simulink model "generic_Truck_And_Trailer"  (R2025a)
settings: Solver=VariableStepAuto  StartTime=0.0  StopTime=350  FixedStep=0.01  MaxStep=0.001  RelTol=1e-3  EnableMultiTasking=on
libraries: TruckMaker4SL x250, simulink x1
(part 10 of 11)

== matlab function generic_Truck_And_Trailer/TruckMaker/Subsystem1/ONE_TRACK_MODEL_TRACTOR_UKF/UKF_ONE_TRACK_TRUCK_AND_TRAILER_WORKING_MODEL  ==
  data: z input; u input; xhat output; Q input; R input; Ts input; P output; dxdt output; innovation output; K_out output; S_out output; z_pred_out output; truck_Ff output; truck_Fr output; trailer_v_hitch output; data input; trailer_v_axle output; trailer_F_hitch output; trailer_F_tire output; truck_v_hitch output
function [xhat, P, dxdt, innovation, K_out, S_out, z_pred_out,truck_Ff,truck_Fr, trailer_v_hitch,trailer_v_axle,trailer_F_hitch,trailer_F_tire,truck_v_hitch] = UKF_TruckTrailer(z,u,Q,R,Ts,data)
persistent x Pk dxdt_old t
%% =========================
%% INIT
%% =========================
if isempty(x)
    x = [15;0.1;0.1;14;14;0;0;5]; % [vx vy wz Cf Cr psi wz_tr Cr_tr]
end
if isempty(Pk)
    Pk = diag([0.1 0.1 0.1 5 5 0.03 0.1 5]);
end
if isempty(dxdt_old)
    dxdt_old = zeros(8,1);
end
if isempty(t)
    t = 0;
end
t = data;
if t < 30
    xhat=x; P=Pk; dxdt=dxdt_old;
    
    innovation=zeros(length(z),1);
    K_out=zeros(length(x), length(z));
    S_out=eye(length(z));
    z_pred_out=zeros(length(z),1);
    
    trailer_v_axle   = zeros(3,1);
    trailer_v_hitch = zeros(3,1);
    truck_Ff = zeros(2,1);
    truck_Fr = zeros(2,1);
    truck_v_hitch=zeros(3,1);
    
    trailer_F_hitch = zeros(2,1);
    trailer_F_tire = zeros(2,1);
    
    return
end
%% =========================
%% CONSTANTS
%% =========================
g = 9.82;
% Truck
m = 6800; 
Jz = 12994.917; 
Rwheel = 0.50;
w_track = 2.1; 
% Trailer
m_tr = 31960;
Jz_tr = 145971.764;
% Geometry & koordinat punkter på Truck
p_cog = [3.473;0;0.925];
p_fax = [4.520;0;0.50];
p_rax = [0.950;0;0.50];
p_imu = [3.600;0;1.000];
hitch = [1.9;0;1.21];
Rcog = p_imu - p_cog;
hHitch= hitch(3);
lf = abs(p_fax(1)-p_cog(1)); 
lr = abs(p_cog(1)-p_rax(1)); 
L = lf + lr;
h = p_cog(3);
Rfax = p_fax - p_cog; Rfax(3)=-p_cog(3);
Rrax = p_rax - p_cog; Rrax(3)=-p_cog(3);
Rhitch = hitch - p_cog;
lhitch = Rhitch(1);
% Geometry Trailer
p_cog_tr = [-6.195;0;1.95];
p_rFax_tr = [-7.75;0;0.5];
p_rMax_tr = [-9.0;0;0.5];
p_rRax_tr = [-10.25;0;0.5];
hitch_tr = [-1.25;0;1.25];

% Avstånd från hitch till trailer-punkter
lf_tr = abs(hitch_tr(1)-p_cog_tr(1));
lr_f_tr = abs(p_cog_tr(1)-p_rFax_tr(1));
lr_m_tr = abs(p_cog_tr(1)-p_rMax_tr(1));
lr_r_tr = abs(p_cog_tr(1)-p_rRax_tr(1));
L_tr = lf_tr + lr_m_tr; % Hävarm till mittaxel

% Vektorer från trailer-CoG till axlar (för cross-product)
Frax_tr = p_rFax_tr - p_cog_tr; Frax_tr(3) = -hitch_tr(3);
Mrax_tr = p_rMax_tr - p_cog_tr; Mrax_tr(3) = -hitch_tr(3);
Rlrax_tr = p_rRax_tr - p_cog_tr; Rlrax_tr(3) =-hitch_tr(3);
Rhitch_tr = hitch_tr - p_cog_tr; Rhitch_tr(3) = -hitch_tr(3);

h_cog_tr = p_cog_tr(3);

%% =========================
%% INPUTS
%% =========================
delta = u(1); 
T_rl = u(2);   
T_rr = u(3);
Fxh = u(4); 
Fx_f_brake  = -abs(u(6)) / Rwheel; 
Fx_r_brake  = -abs(u(7)) / Rwheel;
Fx_vehicle = (T_rl+T_rr)/Rwheel + Fx_r_brake +Fx_f_brake;

%% =========================
%% UKF PARAMS
%% =========================
n = length(x);
nSPx = 2*n+1;
W0 = 1 - n/3;
Wi = (1 - W0)/(2*n);
gamma = sqrt(n/(1 - W0));

%% =========================
%% SIGMA POINTS (PRIOR)
%% =========================
Pk = (Pk+Pk')/2 + 1e-9*eye(n);
Sx = chol(Pk,'lower');
X_pre = zeros(n,nSPx);
X_pre(:,1) = x;
for i=1:n
    X_pre(:,i+1)   = x + gamma*Sx(:,i);
    X_pre(:,i+1+n) = x - gamma*Sx(:,i);
end

%% =========================
%% PREDICTION
%% =========================
X_pred = zeros(n,nSPx);
dxdt_model = zeros(n,1);
truck_Ff = zeros(2,1);
truck_Fr = zeros(2,1);
truck_v_hitch = zeros(3,1);
    
trailer_v_axle = zeros(3,1);
trailer_v_hitch = zeros(3,1);
trailer_F_hitch = zeros(2,1);
trailer_F_tire = zeros(2,1);

for k=1:nSPx
    Xk = X_pre(:,k);
    vx=Xk(1); vy=Xk(2); wz=Xk(3); Cf=Xk(4); Cr=Xk(5);
    psi=Xk(6); wz_tr=Xk(7); Cr_tr=Xk(8);
    
    v_cog=[vx;vy;0];
    omega=[0;0;wz];
    
    %% ===== TRAILER =====
    v_hitch_truck = v_cog + cross(omega,Rhitch);
    
    Rot_tr=[cos(psi) -sin(psi) 0;
            sin(psi) cos(psi)  0; 
              0         0      1];
   
    v_hitch_trailer = Rot_tr.' * v_hitch_truck;
    
    % Beräkna Fz för trailer (Dela på 3 axlar!)
    Fz_hitch = (m_tr*g*lr_m_tr) / (L_tr); 
    Fz_tr_total = m_tr*g - Fz_hitch;
    Fz_tr_each = Fz_tr_total / 3;

    % Hastigheter och slip för traileraxlar (relativt trailer CoG)
    omega_tr = [0;0;wz_tr];
    v_cog_tr = v_hitch_trailer - cross(omega_tr, Rhitch_tr);
    
    v_tr_f = v_cog_tr + cross(omega_tr, Frax_tr);
    v_tr_m = v_cog_tr + cross(omega_tr, Mrax_tr);
    v_tr_r = v_cog_tr + cross(omega_tr, Rlrax_tr);  
    
    alpha_tr_f = atan2(v_tr_f(2), max(abs(v_tr_f(1)), 0.1));
    alpha_tr_m = atan2(v_tr_m(2), max(abs(v_tr_m(1)), 0.1));
    alpha_tr_r = atan2(v_tr_r(2), max(abs(v_tr_r(1)), 0.1));
    
    Fy_f_tr = -Cr_tr * alpha_tr_f * Fz_tr_each;
    Fy_m_tr = -Cr_tr * alpha_tr_m * Fz_tr_each;
    Fy_r_tr = -Cr_tr * alpha_tr_r * Fz_tr_each;
    
    % Hitch-kraft (momentjämvikt kring CoG-punkten)
    Fyh_mod = (Fy_f_tr*lf_tr + Fy_m_tr*lr_m_tr + Fy_r_tr*lr_r_tr) / (lf_tr + lr_m_tr);
 
    if k==1
        trailer_v_hitch = v_hitch_trailer;
        trailer_v_axle = v_tr_m;
        truck_v_hitch = v_hitch_truck;
        trailer_F_hitch = [Fyh_mod; Fz_hitch];
        trailer_F_tire = [Fy_m_tr; Fz_tr_each];
    end

    %% ===== TRUCK =====
    % Transformera hitch-krafter till Truckens system
    F_hitch_body = Rot_tr * [Fxh; Fyh_mod; 0];
    
    Rotf=[cos(delta) -sin(delta)  0; 
          sin(delta)  cos(delta)  0;
              0           0       1];
    vf = Rotf.'*(v_cog + cross(omega,Rfax));
    vr = v_cog + cross(omega,Rrax);
    
    alpha_f = atan2(vf(2),max(abs(vf(1)),0.1));
    alpha_r = atan2(vr(2),max(abs(vr(1)),0.1));
    
    % Vertikallast Truck
    ax_est = (Fx_vehicle - F_hitch_body(1))/m; 
    Ffz = (m*g*lr - m*ax_est*h + Fz_hitch*(hitch(1) - p_rax(1)) - F_hitch_body(1)*hHitch) / L;
    Frz = (m*g*lf + m*ax_est*h + Fz_hitch*(p_fax(1) - hitch(1)) + F_hitch_body(1)*hHitch) / L;
    
    Fy_f = -Cf * alpha_f * Ffz;
    Fy_r = -Cr * alpha_r * Frz;
    
    %% ===== DYNAMICS =====
    dvx = (Fx_vehicle - Fy_f*sin(delta) - F_hitch_body(1))/m + vy*wz;
    dvy = (Fy_f*cos(delta) + Fy_r - F_hitch_body(2))/m - vx*wz;
    dwz = (lf*Fy_f*cos(delta) - lr*Fy_r - lhitch*F_hitch_body(2))/Jz;
    
    dpsi = wz - wz_tr;  % <-- KORRIGERAT TECKEN (wz_tr - wz)
    % Moment kring trailer CoG
    dwz_tr = (lf_tr*Fyh_mod - lr_f_tr*Fy_f_tr - lr_m_tr*Fy_m_tr - lr_r_tr*Fy_r_tr)/Jz_tr;
    
    if k==1
        dxdt_model=[dvx;dvy;dwz;0;0;dpsi;dwz_tr;0];
        truck_Ff = [Fy_f;Ffz];
        truck_Fr = [Fy_r;Frz];
    end
    X_pred(:,k) = Xk + Ts*[dvx; dvy; dwz; 0; 0; dpsi; dwz_tr; 0];
end

%% ===== MEAN & COV
x_pred=zeros(n,1);
for k=1:nSPx
    w=(k==1)*W0+(k>1)*Wi;
    x_pred=x_pred+w*X_pred(:,k);
end
P_pred=zeros(n);
for k=1:nSPx
    w=(k==1)*W0+(k>1)*Wi;
    dx=X_pred(:,k)-x_pred;
    P_pred=P_pred+w*(dx*dx');
end
P_pred=P_pred+Q*Ts;

%% =========================
%% MEASUREMENT UPDATE
%% =========================
Sx=chol((P_pred+P_pred')/2 + 1e-9*eye(n),'lower');
X_post=zeros(n,nSPx);
X_post(:,1)=x_pred;
for i=1:n
    X_post(:,i+1)  =x_pred + gamma*Sx(:,i);
    X_post(:,i+1+n)=x_pred - gamma*Sx(:,i);
end

Z=zeros(10,nSPx);
for k=1:nSPx
    Xk=X_post(:,k);
    vx=Xk(1); vy=Xk(2); wz=Xk(3); Cf=Xk(4); Cr=Xk(5);
    psi=Xk(6); wz_tr=Xk(7); Cr_tr=Xk(8); 
    
    % Beräkna Fz för trailer (samma som i prediction)
    Fz_hitch_meas = (m_tr*g*lr_m_tr) / (L_tr); 
    Fz_tr_total_meas = m_tr*g - Fz_hitch_meas;
    Fz_tr_each_meas = Fz_tr_total_meas / 3;
    
    % Upprepa kraftberäkning för z_pred
    Rot_tr=[cos(psi) -sin(psi) 0;
            sin(psi)  cos(psi) 0;
                0       0      1];

    v_hitch_tr = Rot_tr.' * ([vx;vy;0] + cross([0;0;wz],Rhitch));
    
    % Samma logik som i prediction
    v_cog_tr_meas = v_hitch_tr - cross([0;0;wz_tr], Rhitch_tr);
    v_tr_m_meas = v_cog_tr_meas + cross([0;0;wz_tr], Mrax_tr);
    alpha_tr_m = atan2(v_tr_m_meas(2), max(abs(v_tr_m_meas(1)), 0.1));
    Fy_m_tr_meas = -Cr_tr * alpha_tr_m * Fz_tr_each_meas;
   
    % Beräkna Fy_f_tr och Fy_r_tr för hitch-kraften
    v_tr_f_meas = v_cog_tr_meas + cross([0;0;wz_tr], Frax_tr);
    v_tr_r_meas = v_cog_tr_meas + cross([0;0;wz_tr], Rlrax_tr);
    alpha_tr_f_meas = atan2(v_tr_f_meas(2), max(abs(v_tr_f_meas(1)), 0.1));
    alpha_tr_r_meas = atan2(v_tr_r_meas(2), max(abs(v_tr_r_meas(1)), 0.1));
    Fy_f_tr_meas = -Cr_tr * alpha_tr_f_meas * Fz_tr_each_meas;
    Fy_r_tr_meas = -Cr_tr * alpha_tr_r_meas * Fz_tr_each_meas;
    
    % Hitch-kraft (momentjämvikt)
    Fyh_mod_meas = (Fy_f_tr_meas*lf_tr + Fy_m_tr_meas*lr_m_tr + Fy_r_tr_meas*lr_r_tr) / (lf_tr + lr_m_tr);
    
    F_hitch_body = Rot_tr * [Fxh; Fyh_mod_meas; 0];
    
    % Vertikallast Truck för measurement
    ax_est_meas = (Fx_vehicle - F_hitch_body(1))/m; 
    Ffz_meas = (m*g*lr - m*ax_est_meas*h + Fz_hitch_meas*(hitch(1) - p_rax(1)) - F_hitch_body(1)*hHitch) / L;
    Frz_meas = (m*g*lf + m*ax_est_meas*h + Fz_hitch_meas*(p_fax(1) - hitch(1)) + F_hitch_body(1)*hHitch) / L;
    
    alpha_f = atan2(vy + lf*wz, max(abs(vx),0.1)) - delta;
    alpha_r = atan2(vy - lr*wz, max(abs(vx),0.1));
    Fy_f_meas = -Cf * alpha_f * Ffz_meas;
    Fy_r_meas = -Cr * alpha_r * Frz_meas;
    
    a_spec_x = (Fx_vehicle - Fy_f_meas*sin(delta) - F_hitch_body(1))/m;
    a_spec_y = (Fy_f_meas*cos(delta) + Fy_r_meas - F_hitch_body(2))/m;
    dwz_m = (lf*Fy_f_meas*cos(delta) - lr*Fy_r_meas - lhitch*F_hitch_body(2))/Jz;
    
    a_imu = [a_spec_x; a_spec_y; 0] + cross([0;0;wz],cross([0;0;wz],Rcog)) + cross([0;0;dwz_m],Rcog);
    v_imu = [vx;vy;0] + cross([0;0;wz],Rcog);
    
    Z(:,k)=[a_imu(1:2); v_imu(1); v_imu(2); wz; ...
            (vx - wz*w_track/2)/Rwheel; (vx + wz*w_track/2)/Rwheel; ...
            (v_tr_m_meas(1) - wz_tr*w_track/2)/Rwheel; (v_tr_m_meas(1) + wz_tr*w_track/2)/Rwheel; Fyh_mod_meas];
end

z_pred=zeros(10,1);
for k=1:nSPx
    w=(k==1)*W0+(k>1)*Wi;
    z_pred=z_pred+w*Z(:,k);
end

valid_idx = ~isnan(z);
z_used = z(valid_idx);
z_pred_used = z_pred(valid_idx);
R_used = R(valid_idx,valid_idx);

S_cov=zeros(length(z_used));
Pxz=zeros(n,length(z_used));
for k=1:nSPx
    w=(k==1)*W0+(k>1)*Wi;
    dz=Z(valid_idx,k)-z_pred_used;
    dx=X_post(:,k)-x_pred;
    S_cov=S_cov+w*(dz*dz');
    Pxz=Pxz+w*(dx*dz');
end
S_cov=S_cov+R_used;
K=Pxz/S_cov;

x=x_pred + K*(z_used - z_pred_used);
Pk=P_pred - K*S_cov*K';
Pk=(Pk+Pk')/2 + 1e-9*eye(n);

%% OUTPUT
xhat=x; P=Pk; dxdt=dxdt_model;
innovation=zeros(length(z),1); innovation(valid_idx)=z_used - z_pred_used;
K_out=zeros(n,length(z)); K_out(:,valid_idx)=K;
S_out=zeros(length(z)); S_out(valid_idx,valid_idx)=S_cov;
z_pred_out=z_pred;

end

== matlab function generic_Truck_And_Trailer/TruckMaker/Two_TRack_Model/MATLAB Function1 ==
  data: z input; u input; xhat output; Q input; R input; Ts input; P output
function [xhat, P] = CKF_Bicycle_IPG(z, u, Q, R, Ts)
% Cubature Kalman Filter for One-Track vehicle model
% States: [vx vy r Cf Cr]'
% Measurements: [ay r vx]'

% -------------------------------------------------
% Persistent states (SIMULINK SAFE)
% -------------------------------------------------
persistent x Pk

if isempty(x)
    x  = [15; 0; 0.05; 6e4; 6e4];
    Pk = diag([1 1 0.05 2e4 2e4].^2);
end

n = length(x);   % state dimension
m = length(z);   % measurement dimension

% -------------------------------------------------
% Cubature points
% -------------------------------------------------
Xi = sqrt(n) * [eye(n) -eye(n)];
W  = ones(1,2*n) / (2*n);

% -------------------------------------------------
% PREDICTION STEP
% -------------------------------------------------
X_pred = zeros(n,2*n);
S = chol(Pk,'lower');

for i = 1:2*n
    X_sigma = x + S*Xi(:,i);
    X_pred(:,i) = VehicleDynamics(X_sigma, u, Ts);
end

x_pred = X_pred * W';

P_pred = Q;
for i = 1:2*n
    dx = X_pred(:,i) - x_pred;
    P_pred = P_pred + W(i) * (dx*dx');
end

% -------------------------------------------------
% MEASUREMENT PREDICTION
% -------------------------------------------------
Z_sigma = zeros(m,2*n);
for i = 1:2*n
    Z_sigma(:,i) = MeasurementModel(X_pred(:,i), u);
end

z_pred = Z_sigma * W';

Pzz = R;
Pxz = zeros(n,m);
for i = 1:2*n
    dz = Z_sigma(:,i) - z_pred;
    dx = X_pred(:,i) - x_pred;
    Pzz = Pzz + W(i)*(dz*dz');
    Pxz = Pxz + W(i)*(dx*dz');
end

% -------------------------------------------------
% UPDATE STEP
% -------------------------------------------------
K = Pxz / Pzz;

x  = x_pred + K*(z - z_pred);
Pk = P_pred - K*Pzz*K';

xhat = x;
P    = Pk;

end
function x_next = VehicleDynamics(x, u, Ts)

% States
vx = x(1); vy = x(2); r = x(3);
Cf = x(4); Cr = x(5);

% Inputs
delta = u(1);    % steering angle [rad]
Fx    = u(2);    % longitudinal force [N]

% Vehicle parameters
m  = 7000;
Jz = 14232;
lf = 1.12;
lr = 2.45;

vx_eff = max(abs(vx), 3);

% Slip angles
alpha_f = (vy + lf*r)/vx_eff - delta;
alpha_r = (vy - lr*r)/vx_eff;

% Tire forces
Fyf = -Cf * alpha_f;
Fyr = -Cr * alpha_r;

% Dynamics
dvx = (Fx - Fyf*sin(delta) + vy*r)/m;
dvy = (Fyf*cos(delta) + Fyr - vx*r)/m;
dr  = (lf*Fyf*cos(delta) - lr*Fyr)/Jz;

% Parameters as random walk
dCf = 0;
dCr = 0;

% Euler integration
x_next = x + Ts*[dvx; dvy; dr; dCf; dCr];

end
function z = MeasurementModel(x, u)

vx = x(1); vy = x(2); r = x(3);
Cf = x(4); Cr = x(5);
delta = u(1);

% Vehicle parameters
m  = 7000;
lf = 1.12;
lr = 2.45;

vx_eff = max(abs(vx),3);

% Slip angles
alpha_f = (vy + lf*r)/vx_eff - delta;
alpha_r = (vy - lr*r)/vx_eff;

% Tire forces
Fyf = -Cf * alpha_f;
Fyr = -Cr * alpha_r;

% Lateral acceleration (IMU)
dvy = (Fyf*cos(delta) + Fyr - vx*r)/m;
ay  = dvy + vx*r;

% Measurement vector
z = [
    ay
    r
    vx
];

end

== matlab function generic_Truck_And_Trailer/TruckMaker/Subsystem1/Subsystem_Noisey Measurements/MATLAB Function5 ==
  data: truth input; vel_meas output
function vel_meas = imu_vel_noise(truth)
    

sigma = 0.05; % m/s^2 (tune later)

vel_meas = truth + sigma * randn(size(truth));


end

== matlab function generic_Truck_And_Trailer/TruckMaker/Subsystem1/ONE_TRACK_MODEL_TRACTOR_UKF/MATLAB Function3 ==
  data: vx_tire input; TCS_trailer output; vy_tire input; Fy_tire input; Fz_tire input; SSA output
function  [TCS_trailer,SSA]= fcn(vx_tire,vy_tire,Fy_tire,Fz_tire)
SSA=atan2(vy_tire,max(abs(vx_tire),0.1));
TCS_trailer = Fy_tire/(SSA*Fz_tire) ;

== matlab function generic_Truck_And_Trailer/TruckMaker/Subsystem1/ONE_TRACK_MODEL_TRACTOR_UKF/UKF_ONE_TRACK3 ==
  data: z input; u input; xhat output; Q input; R input; Ts input; P output; dxdt output; innovation output; K_out output; S_out output; z_pred_out output; data input; truck_Ff output; truck_Fr output; trailer_v_hitch output; trailer_v_axle output; trailer_F_hitch output; trailer_F_tire output; truck_v_hitch output
function [xhat, P, dxdt, innovation, K_out, S_out, z_pred_out,truck_Ff,truck_Fr, trailer_v_hitch,trailer_v_axle,trailer_F_hitch,trailer_F_tire,truck_v_hitch] = UKF_TruckTrailer(z,u,Q,R,Ts,data)
persistent x Pk dxdt_old t
%% =========================
%% INIT
%% =========================
if isempty(x)
    x = [15;0.1;0.1;14;14;0;0;14]; % [vx vy wz Cf Cr psi wz_tr Cr_tr]
end
if isempty(Pk)
    Pk = diag([0.1 0.1 0.1 5 5 0.03 0.1 5]);
end
if isempty(dxdt_old)
    dxdt_old = zeros(8,1);
end
if isempty(t)
    t = 0;
end
t = data;
if t < 30
    xhat=x; P=Pk; dxdt=dxdt_old;
    
    innovation=zeros(length(z),1);
    K_out=zeros(length(x), length(z));
    S_out=eye(length(z));
    z_pred_out=zeros(length(z),1);
    
    trailer_v_axle   = zeros(3,1);
    trailer_v_hitch = zeros(3,1);
    truck_Ff = zeros(2,1);
    truck_Fr = zeros(2,1);
    truck_v_hitch=zeros(3,1);
    
    trailer_F_hitch = zeros(2,1);
    trailer_F_tire = zeros(2,1);
    
    return
end
%% =========================
%% CONSTANTS
%% =========================
g = 9.82;
% Truck
m = 6800; 
Jz = 12994.917; 
Rwheel = 0.50;
w_track = 2.1; 
% Trailer
m_tr = 31960;
Jz_tr = 145971.764;
% Geometry & koordinat punkter på Truck
p_cog = [3.473;0;0.925];
p_fax = [4.520;0;0.50];
p_rax = [0.950;0;0.50];
p_imu = [3.600;0;1.000];
hitch = [1.9;0;1.21];
Rcog = p_imu - p_cog;
hHitch= hitch(3);
lf = abs(p_fax(1)-p_cog(1)); 
lr = abs(p_cog(1)-p_rax(1)); 
L = lf + lr;
h = p_cog(3);
Rfax = p_fax - p_cog; Rfax(3)=-p_cog(3);
Rrax = p_rax - p_cog; Rrax(3)=-p_cog(3);
Rhitch = hitch - p_cog;
lhitch = Rhitch(1);
% Geometry Trailer
p_cog_tr = [-6.195;0;1.95];
p_rFax_tr = [-7.75;0;0.5];
p_rMax_tr = [-9.0;0;0.5];
p_rRax_tr = [-10.25;0;0.5];
hitch_tr = [-1.25;0;1.25];

% Avstånd från hitch till trailer-punkter
lf_tr = abs(hitch_tr(1)-p_cog_tr(1));
lr_f_tr = abs(p_cog_tr(1)-p_rFax_tr(1));
lr_m_tr = abs(p_cog_tr(1)-p_rMax_tr(1));
lr_r_tr = abs(p_cog_tr(1)-p_rRax_tr(1));
L_tr = lf_tr + lr_m_tr; % Hävarm till mittaxel

% Vektorer från trailer-CoG till axlar (för cross-product)
Frax_tr = p_rFax_tr - p_cog_tr; Frax_tr(3) = 0;
Mrax_tr = p_rMax_tr - p_cog_tr; Mrax_tr(3) = 0;
Rlrax_tr = p_rRax_tr - p_cog_tr; Rlrax_tr(3) = 0;
Rhitch_tr = hitch_tr - p_cog_tr; Rhitch_tr(3) = 0;

h_tr = p_cog_tr(3);

%% =========================
%% INPUTS
%% =========================
delta = u(1); 
T_rl = u(2);   
T_rr = u(3);
Fxh = u(4); 
Fx_f_brake  = -abs(u(6)) / Rwheel; 
Fx_r_brake  = -abs(u(7)) / Rwheel;
Fx_vehicle = (T_rl+T_rr)/Rwheel + Fx_r_brake +Fx_f_brake;

%% =========================
%% UKF PARAMS
%% =========================
n = length(x);
nSPx = 2*n+1;
W0 = 1 - n/3;
Wi = (1 - W0)/(2*n);
gamma = sqrt(n/(1 - W0));

%% =========================
%% SIGMA POINTS (PRIOR)
%% =========================
Pk = (Pk+Pk')/2 + 1e-9*eye(n);
Sx = chol(Pk,'lower');
X_pre = zeros(n,nSPx);
X_pre(:,1) = x;
for i=1:n
    X_pre(:,i+1)   = x + gamma*Sx(:,i);
    X_pre(:,i+1+n) = x - gamma*Sx(:,i);
end

%% =========================
%% PREDICTION
%% =========================
X_pred = zeros(n,nSPx);
dxdt_model = zeros(n,1);
truck_Ff = zeros(2,1);          % <--- FIX
truck_Fr = zeros(2,1);          % <--- FIX
truck_v_hitch = zeros(3,1);     % <--- FIX
    
trailer_v_axle = zeros(3,1);    % <--- FIX
trailer_v_hitch = zeros(3,1);   % <--- FIX
trailer_F_hitch = zeros(2,1);   % <--- FIX
trailer_F_tire = zeros(2,1);    % <--- FIX

for k=1:nSPx
    Xk = X_pre(:,k);
    vx=Xk(1); vy=Xk(2); wz=Xk(3); Cf=Xk(4); Cr=Xk(5);
    psi=Xk(6); wz_tr=Xk(7); Cr_tr=Xk(8);
    
    v_cog=[vx;vy;0];
    omega=[0;0;wz];
    
    %% ===== TRAILER =====
    v_hitch_truck = v_cog + cross(omega,Rhitch);
    Rot_tr=[cos(psi) -sin(psi) 0; sin(psi) cos(psi) 0; 0 0 1];
    v_hitch_trailer = Rot_tr.' * v_hitch_truck;
    
    % Beräkna Fz för trailer (Dela på 3 axlar!)
    Fz_hitch = (m_tr*g*lr_m_tr) / (lf_tr + lr_m_tr); 
    Fz_tr_total = (m_tr*g - Fz_hitch);
    Fz_tr_each = Fz_tr_total / 3;

    % Hastigheter och slip för traileraxlar (relativt trailer CoG)
    % Vi förenklar: v_cog_tr = v_hitch_trailer - cross(omega_tr, Rhitch_tr)
    omega_tr = [0;0;wz_tr];
    v_cog_tr = v_hitch_trailer - cross(omega_tr, Rhitch_tr);
    
    v_tr_f = v_cog_tr + cross(omega_tr, Frax_tr);
    v_tr_m = v_cog_tr + cross(omega_tr, Mrax_tr);
    v_tr_r = v_cog_tr + cross(omega_tr, Rlrax_tr);
    
    alpha_tr_f = atan2(v_tr_f(2), max(abs(v_tr_f(1)), 0.1));
    alpha_tr_m = atan2(v_tr_m(2), max(abs(v_tr_m(1)), 0.1));
    alpha_tr_r = atan2(v_tr_r(2), max(abs(v_tr_r(1)), 0.1));
    
    Fy_f_tr = -Cr_tr * alpha_tr_f * Fz_tr_each;
    Fy_m_tr = -Cr_tr * alpha_tr_m * Fz_tr_each;
    Fy_r_tr = -Cr_tr * alpha_tr_r * Fz_tr_each;
    
    % Hitchkraft (baserad på acceleration i y)
    Fyh_mod = m_tr*(v_hitch_trailer(2)*wz) - (Fy_f_tr + Fy_m_tr + Fy_r_tr);
 
    if k==1
        trailer_v_hitch = v_hitch_trailer;
        trailer_v_axle = v_tr_m;
        truck_v_hitch = v_hitch_truck;
        trailer_F_hitch = [Fyh_mod; Fz_hitch];
        trailer_F_tire = [Fy_m_tr; Fz_tr_each];
    end

    %% ===== TRUCK =====
    % Transformera hitch-krafter till Truckens system (Viktigt för dvx!)
    F_hitch_body = Rot_tr * [Fxh; Fyh_mod; 0];
    
    Rotf=[cos(delta) -sin(delta) 0; sin(delta) cos(delta) 0; 0 0 1];
    vf = Rotf.'*(v_cog + cross(omega,Rfax));
    vr = v_cog + cross(omega,Rrax);
    
    alpha_f = atan2(vf(2),max(abs(vf(1)),0.1));
    alpha_r = atan2(vr(2),max(abs(vr(1)),0.1));
    
    % Vertikallast Truck
    ax_est = (Fx_vehicle - F_hitch_body(1))/m; 
    Ffz = (m*g*lr - m*ax_est*h + Fz_hitch*(hitch(1) - p_rax(1)) - F_hitch_body(1)*hHitch) / L;
    Frz = (m*g*lf + m*ax_est*h + Fz_hitch*(p_fax(1) - hitch(1)) + F_hitch_body(1)*hHitch) / L;
    
    Fy_f = -Cf*alpha_f*Ffz;
    Fy_r = -Cr*alpha_r*Frz;
    
    %% ===== DYNAMICS =====
    dvx = (Fx_vehicle - Fy_f*sin(delta) - F_hitch_body(1))/m + vy*wz;
    dvy = (Fy_f*cos(delta) + Fy_r - F_hitch_body(2))/m - vx*wz;
    dwz = (lf*Fy_f*cos(delta) - lr*Fy_r - lhitch*F_hitch_body(2))/Jz;
    
    dpsi = wz - wz_tr; 
    % Moment kring trailer CoG
    dwz_tr = (lf_tr*Fyh_mod - lr_f_tr*Fy_f_tr - lr_m_tr*Fy_m_tr - lr_r_tr*Fy_r_tr)/Jz_tr;
    
    if k==1
        dxdt_model=[dvx;dvy;dwz;0;0;dpsi;dwz_tr;0];
        truck_Ff = [Fy_f;Ffz];
        truck_Fr = [Fy_r;Frz];
    end
    X_pred(:,k) = Xk + Ts*[dvx; dvy; dwz; 0; 0; dpsi; dwz_tr; 0];
end

%% ===== MEAN & COV
x_pred=zeros(n,1);
for k=1:nSPx
    w=(k==1)*W0+(k>1)*Wi;
    x_pred=x_pred+w*X_pred(:,k);
end
P_pred=zeros(n);
for k=1:nSPx
    w=(k==1)*W0+(k>1)*Wi;
    dx=X_pred(:,k)-x_pred;
    P_pred=P_pred+w*(dx*dx');
end
P_pred=P_pred+Q*Ts;

%% =========================
%% MEASUREMENT UPDATE
%% =========================
Sx=chol((P_pred+P_pred')/2 + 1e-9*eye(n),'lower');
X_post=zeros(n,nSPx);
X_post(:,1)=x_pred;
for i=1:n
    X_post(:,i+1)  =x_pred + gamma*Sx(:,i);
    X_post(:,i+1+n)=x_pred - gamma*Sx(:,i);
end

Z=zeros(10,nSPx);
for k=1:nSPx
    Xk=X_post(:,k);
    vx=Xk(1); vy=Xk(2); wz=Xk(3); Cf=Xk(4); Cr=Xk(5);
    psi=Xk(6); wz_tr=Xk(7); Cr_tr=Xk(8); 
    
    % Upprepa kraftberäkning för z_pred
    Rot_tr=[cos(psi) -sin(psi) 0; sin(psi) cos(psi) 0; 0 0 1];
    v_hitch_tr = Rot_tr.' * ([vx;vy;0] + cross([0;0;wz],Rhitch));
    
    % Samma logik som i prediction
    alpha_tr_m = atan2(v_hitch_tr(2) - lr_m_tr*wz_tr, max(abs(v_hitch_tr(1)),0.1));
    Fy_m_tr = -Cr_tr*alpha_tr_m*Fz_tr_each;
    Fyh_mod = m_tr*(v_hitch_tr(2)*wz) - 3*Fy_m_tr; 
    
    F_hitch_body = Rot_tr * [Fxh; Fyh_mod; 0];
    
    alpha_f = atan2(vy + lf*wz, max(abs(vx),0.1)) - delta;
    alpha_r = atan2(vy - lr*wz, max(abs(vx),0.1));
    Fy_f = -Cf*alpha_f*Ffz;
    Fy_r = -Cr*alpha_r*Frz;
    
    a_spec_x = (Fx_vehicle - Fy_f*sin(delta) - F_hitch_body(1))/m;
    a_spec_y = (Fy_f*cos(delta) + Fy_r - F_hitch_body(2))/m;
    dwz_m = (lf*Fy_f*cos(delta) - lr*Fy_r - lhitch*F_hitch_body(2))/Jz;
    
    a_imu = [a_spec_x; a_spec_y; 0] + cross([0;0;wz],cross([0;0;wz],Rcog)) + cross([0;0;dwz_m],Rcog);
    v_imu = [vx;vy;0] + cross([0;0;wz],Rcog);
    
    Z(:,k)=[a_imu(1:2); v_imu(1); v_imu(2); wz; ...
            (vx - wz*w_track/2)/Rwheel; (vx + wz*w_track/2)/Rwheel; ...
            (vx - wz_tr*w_track/2)/Rwheel; (vx + wz_tr*w_track/2)/Rwheel; Fyh_mod];
end

z_pred=zeros(10,1);
for k=1:nSPx
    w=(k==1)*W0+(k>1)*Wi;
    z_pred=z_pred+w*Z(:,k);
end

valid_idx = ~isnan(z);
z_used = z(valid_idx);
z_pred_used = z_pred(valid_idx);
R_used = R(valid_idx,valid_idx);

S_cov=zeros(length(z_used));
Pxz=zeros(n,length(z_used));
for k=1:nSPx
    w=(k==1)*W0+(k>1)*Wi;
    dz=Z(valid_idx,k)-z_pred_used;
    dx=X_post(:,k)-x_pred;
    S_cov=S_cov+w*(dz*dz');
    Pxz=Pxz+w*(dx*dz');
end
S_cov=S_cov+R_used;
K=Pxz/S_cov;

x=x_pred + K*(z_used - z_pred_used);
Pk=P_pred - K*S_cov*K';
Pk=(Pk+Pk')/2 + 1e-9*eye(n);

%% OUTPUT
xhat=x; P=Pk; dxdt=dxdt_model;
innovation=zeros(length(z),1); innovation(valid_idx)=z_used - z_pred_used;
K_out=zeros(n,length(z)); K_out(:,valid_idx)=K;
S_out=zeros(length(z)); S_out(valid_idx,valid_idx)=S_cov;
z_pred_out=z_pred;

end

== matlab function generic_Truck_And_Trailer/TruckMaker/Subsystem1/ONE_TRACK_MODEL_TRACTOR_UKF/UKF_ONE_TRACK4 ==
  data: z input; u input; xhat output; Q input; R input; Ts input; P output; dxdt output; innovation output; K_out output; S_out output; z_pred_out output; data input; truck_Ff output; truck_Fr output; trailer_v_hitch output; trailer_v_axle output; trailer_F_hitch output; trailer_F_tire output; truck_v_hitch output
function [xhat, P, dxdt, innovation, K_out, S_out, z_pred_out,truck_Ff,truck_Fr, trailer_v_hitch,trailer_v_axle,trailer_F_hitch,trailer_F_tire,truck_v_hitch] = UKF_TruckTrailer(z,u,Q,R,Ts,data)
persistent x Pk dxdt_old t
%% =========================
%% INIT
%% =========================
if isempty(x)
    x = [15;0.1;0.1;7.5;7.5;0;0;4]; % [vx vy wz Cf Cr psi wz_tr Cr_tr]
end
if isempty(Pk)
    Pk = diag([0.1 0.1 0.1 5 5 0.03 0.1 5]);
end
if isempty(dxdt_old)
    dxdt_old = zeros(8,1);
end
if isempty(t)
    t = 0;
end
t = data;
if t < 30
    xhat=x; P=Pk; dxdt=dxdt_old;
    
    innovation=zeros(length(z),1);
    K_out=zeros(length(x), length(z));
    S_out=eye(length(z));
    z_pred_out=zeros(length(z),1);
    
    trailer_v_axle   = zeros(3,1);
    trailer_v_hitch = zeros(3,1);
    truck_Ff = zeros(2,1);
    truck_Fr = zeros(2,1);
    truck_v_hitch=zeros(3,1);
    
    %% Normal Forces 
    trailer_F_hitch = zeros(2,1);
    trailer_F_tire = zeros(2,1);
    
    return
end
%% =========================
%% CONSTANTS
%% =========================
g = 9.82;
% Truck
m = 6800; 
Jz = 12994.917; 
Rwheel = 0.50;
w_track = 2.1; 
% Trailer
m_tr = 31960;
Jz_tr = 145971.764;
% Geometry & koordinat punkter på Truck
p_cog = [3.473;0;0.925];
p_fax = [4.520;0;0.50];
p_rax = [0.950;0;0.50];
p_imu = [3.600;0;1.000];
hitch = [1.9;0;1.21];
Rcog = p_imu - p_cog;
hHitch= hitch(3);
lf = abs(p_fax(1)-p_cog(1)); 
lr = abs(p_cog(1)-p_rax(1)); 
L = lf + lr;
h = p_cog(3);
Rfax = p_fax - p_cog; Rfax(3)=-p_cog(3);
Rrax = p_rax - p_cog; Rrax(3)=-p_cog(3);
Rhitch = hitch - p_cog;
lhitch = Rhitch(1);
%lfhitch = abs(p_fax(1) -hitch(1));

% Geometry Trailer
p_cog_tr = [-6.195;0;1.95];
p_rFax_tr = [-7.75;0;0.5];
p_rMax_tr = [-9.0;0;0.5];
p_rRax_tr = [-10.25;0;0.5];
hitch_tr = [-1.25;0;1.25];

% Avstånd från hitch till trailer-punkter
lf_tr = abs(hitch_tr(1)-p_cog_tr(1));
lr_f_tr = abs(p_cog_tr(1)-p_rFax_tr(1));
lr_m_tr = abs(p_cog_tr(1)-p_rMax_tr(1));
lr_r_tr = abs(p_cog_tr(1)-p_rRax_tr(1));
L_tr = lf_tr + lr_r_tr;

% Vektorer från trailer-CoG till axlar (för cross-product)
Frax_tr = p_rFax_tr - hitch_tr; Frax_tr(3)=-hitch_tr(3);
Mrax_tr = p_rMax_tr - hitch_tr; Mrax_tr(3)=-hitch_tr(3);
Rlrax_tr = p_rRax_tr - hitch_tr; Rlrax_tr(3)=-hitch_tr(3);
h_tr = p_cog_tr(3);
%% =========================
%% INPUTS
%% =========================
delta = u(1); 
T_rl = u(2);   
T_rr = u(3);
Fxh = u(4); 
%Fyh = u(5)*0; 
Fx_f_brake  = -abs(u(6)) / Rwheel; 
Fx_r_brake  = -abs(u(7)) / Rwheel;
%Fx_tr_brake = -abs(u(8)) / Rwheel;
Fx_vehicle = (T_rl+T_rr)/Rwheel + Fx_r_brake +Fx_f_brake;
%% =========================
%% UKF PARAMS
%% =========================
n = length(x);
nSPx = 2*n+1;
W0 = 1 - n/3;
Wi = (1 - W0)/(2*n);
gamma = sqrt(n/(1 - W0));
%% =========================
%% SIGMA POINTS (PRIOR)
%% =========================
Pk = (Pk+Pk')/2 + 1e-9*eye(n);
Sx = chol(Pk,'lower');
X_pre = zeros(n,nSPx);
X_pre(:,1) = x;
for i=1:n
    X_pre(:,i+1)   = x + gamma*Sx(:,i);
    X_pre(:,i+1+n) = x - gamma*Sx(:,i);
end
%% =========================
%% PREDICTION
%% =========================
X_pred = zeros(n,nSPx);
dxdt_model = zeros(n,1);
truck_Ff = zeros(2,1);
truck_Fr = zeros(2,1);
truck_v_hitch=zeros(3,1);
%%Trailer data
trailer_v_axle   = zeros(3,1);
trailer_v_hitch = zeros(3,1);
trailer_F_hitch = zeros(2,1);
trailer_F_tire = zeros(2,1);
for k=1:nSPx
    Xk = X_pre(:,k);
    vx=Xk(1); vy=Xk(2); wz=Xk(3);Cf=Xk(4); Cr=Xk(5);
    
    psi=Xk(6); wz_tr=Xk(7); Cr_tr=Xk(8);
    
    v_cog=[vx;vy;0];
    omega=[0;0;wz];
    
    %% ===== TRAILER =====
    v_hitch_truck = v_cog + cross(omega,Rhitch);
    
    Rot_tr=[cos(psi)  sin(psi) 0;
            -sin(psi) cos(psi)  0;
            0           0      1];
    omega_tr=[0;0;wz_tr];
    
    ax_tr = Fxh/m_tr;

    v_hitch_trailer = Rot_tr * v_hitch_truck;
    
    v_tr_f = v_hitch_trailer + cross(omega_tr, Frax_tr);
    v_tr_m = v_hitch_trailer + cross(omega_tr,Mrax_tr);
    v_tr_r = v_hitch_trailer + cross(omega_tr, Rlrax_tr);

    
    alpha_tr_f = atan2(v_tr_f(2), max(abs(v_tr_f(1)), 0.1));
    alpha_tr_m = atan2(v_tr_m(2),max(abs(v_tr_m(1)),0.1));
    alpha_tr_r = atan2(v_tr_r(2), max(abs(v_tr_r(1)), 0.1));
    
    
   
    
    Fz_hitch = (m_tr*g*lr_r_tr/L_tr - m_tr*ax_tr*(h_tr-hHitch)/L_tr);
    Fz_tr    = (m_tr*g - Fz_hitch)/3;

    Fy_f_tr = -Cr_tr * alpha_tr_f * Fz_tr;
    Fy_m_tr = -Cr_tr* alpha_tr_m * Fz_tr;
    Fy_r_tr = -Cr_tr * alpha_tr_r * Fz_tr;
    
    %+ lm_tr*Fym_tr
    % Beräknar modellens sidkraft för hitch
    Fyh_mod = (lr_m_tr * Fy_m_tr  + lr_f_tr * Fy_f_tr + lr_r_tr * Fy_r_tr) / lf_tr;
 
    if k==1
        trailer_v_hitch = v_hitch_trailer;
        trailer_v_axle=v_tr_m;
        
        truck_v_hitch=v_hitch_truck;
        trailer_F_hitch = [Fyh_mod;Fz_hitch];
        trailer_F_tire = [Fy_m_tr;Fz_tr];
    end
    %% ===== TRUCK =====
    Rotf=[cos(delta) -sin(delta) 0;
          sin(delta) cos(delta)  0; 
              0            0     1];
    vf = Rotf.'*(v_cog + cross(omega,Rfax));
    vr = v_cog + cross(omega,Rrax);
    
    alpha_f = atan2(vf(2),max(abs(vf(1)),0.1));
    alpha_r = atan2(vr(2),max(abs(vr(1)),0.1));
    
    F_hitch_trailer=[u(4); Fyh_mod; 0];
    F_hitch_body= Rot_tr.' * F_hitch_trailer;
    ax_est = (Fx_vehicle - F_hitch_body(1))/m; 
    
    %Ffz = (m*g*lr - m*ax_est*(h-hHitch) + Fz_hitch*(hitch(1) - p_rax(1)) ) / L; %- F_hitch_body(1)*hHitch
    %Frz = (m*g*lf + m*ax_est*(h-hHitch) + Fz_hitch*(p_fax(1) - hitch(1)) ) / L; %+ F_hitch_body(1)*hHitch
    
    Ffz = (m*g*lr - m*ax_est*h + Fz_hitch*(hitch(1) - p_rax(1)) - F_hitch_body(1)*hHitch) / L;
    Frz = (m*g*lf + m*ax_est*h + Fz_hitch*(p_fax(1) - hitch(1)) + F_hitch_body(1)*hHitch) / L;
    Fy_f = -Cf*alpha_f*Ffz;
    Fy_r = -Cr*alpha_r*Frz;
    
    %% ===== DYNAMICS =====
    dvx = (Fx_vehicle - Fy_f*sin(delta) - F_hitch_body(1))/m + vy*wz;
    dvy = (Fy_f*cos(delta) + Fy_r - F_hitch_body(2))/m - vx*wz;
    dwz = (lf*Fy_f*cos(delta) - lr*Fy_r - lhitch*(F_hitch_body(2)))/Jz;
    dpsi = wz - wz_tr; 
    
    ay_hitch_truck = (Fy_f*cos(delta) + Fy_r - F_hitch_body(2))/m; % Truckens acceleration
    Fyh_mod = m_tr * (ay_hitch_truck) - (Fy_f_tr + Fy_m_tr + Fy_r_tr);
    % --- ÄNDRING HÄR FÖR ATT FIXA OFFSET ---
   
    %dwz_tr = (-lr_r_tr*Fy_m_tr + lf_tr*Fyh_mod )/Jz_tr;
    %dwz_tr = (lf_tr*Fyh_mod - lr_f_tr*Fy_f_tr - lr_m_tr*Fy_m_tr - lr_r_tr*Fy_r_tr)/Jz_tr;
    %dwz_tr = (lf_tr * Fyh_mod - (lr_f_tr * Fy_f_tr + lr_m_tr * Fy_m_tr + lr_r_tr * Fy_r_tr)) / Jz_tr;
    dwz_tr = (lf_tr*Fyh_mod - lr_f_tr*Fy_f_tr - lr_m_tr*Fy_m_tr - lr_r_tr*Fy_r_tr)/Jz_tr;
    % ---------------------------------------
    
    if k==1
        dxdt_model=[dvx;dvy;dwz;0;0;dpsi;dwz_tr;0];
        truck_Ff = [Fy_f;Ffz];
        truck_Fr =  [Fy_r;Frz];
    end
    X_pred(:,k) = Xk + Ts*[dvx; dvy; dwz; 0; 0; dpsi; dwz_tr; 0];
end
%% ===== MEAN & COV
x_pred=zeros(n,1);
P_pred=zeros(n);
for k=1:nSPx
    w=(k==1)*W0+(k>1)*Wi;
    x_pred=x_pred+w*X_pred(:,k);
end
for k=1:nSPx
    w=(k==1)*W0+(k>1)*Wi;
    dx=X_pred(:,k)-x_pred;
    P_pred=P_pred+w*(dx*dx');
end
P_pred=P_pred+Q*Ts;
%% =========================
%% MEASUREMENT
%% =========================
Sx=chol((P_pred+P_pred')/2 + 1e-9*eye(n),'lower');
X_post=zeros(n,nSPx);
X_post(:,1)=x_pred;
for i=1:n
    X_post(:,i+1)  =x_pred + gamma*Sx(:,i);
    X_post(:,i+1+n)=x_pred - gamma*Sx(:,i);
end
Z=zeros(10,nSPx); % Fixat till 10 rader
for k=1:nSPx
    Xk=X_post(:,k);
    vx=Xk(1); vy=Xk(2); wz=Xk(3); Cf=Xk(4); Cr=Xk(5);
    psi=Xk(6); wz_tr=Xk(7); Cr_tr=Xk(8); 
    
    v_cog=[vx;vy;0]; omega=[0;0;wz];
    Rot_tr=[cos(psi) sin(psi) 0;
            -sin(psi)  cos(psi) 0;  
                0         0    1];
    omega_tr=[0;0;wz_tr];
    % v_hitch_tr = Rot_tr.' * (v_cog + cross(omega,Rhitch));
    % v_tr_m = v_hitch_tr + cross(omega_tr,Mrax_tr);
    % alpha_tr_m = atan2(v_tr_m(2),max(abs(v_tr_m(1)),0.1));
    % ax_tr = Fxh / m_tr; 
    % 
    % Fz_hitch = (m_tr*g*lr_r_tr/L_tr - m_tr*ax_tr*(h_tr-hHitch)/L_tr);
    % Fy_m_tr = -Cr_tr*alpha_tr_m*(m_tr*g - Fz_hitch);
    % Fyh_mod = (lr_m_tr * Fy_m_tr) / lf_tr; 

    ax_tr = Fxh/m_tr;

    v_hitch_trailer = Rot_tr * v_hitch_truck;
    
    v_tr_f = v_hitch_trailer + cross(omega_tr, Frax_tr);
    v_tr_m = v_hitch_trailer + cross(omega_tr,Mrax_tr);
    v_tr_r = v_hitch_trailer + cross(omega_tr, Rlrax_tr);

    alpha_tr_f = atan2(v_tr_f(2), max(abs(v_tr_f(1)), 0.1));
    alpha_tr_m = atan2(v_tr_m(2),max(abs(v_tr_m(1)),0.1));
    alpha_tr_r = atan2(v_tr_r(2), max(abs(v_tr_r(1)), 0.1));
    
    Fz_hitch = (m_tr*g*lr_r_tr/L_tr - m_tr*ax_tr*(h_tr-hHitch)/L_tr);
    Fz_tr    = (m_tr*g - Fz_hitch)/3;

    Fy_f_tr = -Cr_tr * alpha_tr_f * Fz_tr;
    Fy_m_tr = -Cr_tr* alpha_tr_m * Fz_tr;
    Fy_r_tr = -Cr_tr * alpha_tr_r * Fz_tr;
    
    %+ lm_tr*Fym_tr
    % Beräknar modellens sidkraft för hitch
    Fyh_mod = (lr_m_tr * Fy_m_tr  + lr_f_tr * Fy_f_tr + lr_r_tr * Fy_r_tr) / lf_tr;
    
    
    Rotf=[cos(delta) -sin(delta) 0; 
          sin(delta)  cos(delta) 0; 
              0           0      1];
    vf = Rotf.'*(v_cog + cross(omega,Rfax));
    alpha_f = atan2(vf(2),max(abs(vf(1)),0.1));
    alpha_r = atan2(vy - lr*wz, max(abs(vx),0.1));
    
    F_hitch_body= Rot_tr.'* [u(4); Fyh_mod; 0];
    ax_est = (Fx_vehicle - F_hitch_body(1))/m;
    %Ffz = (m*g*lr - m*ax_est*(h-hHitch) + Fz_hitch*(hitch(1) - p_rax(1)) ) / L; %- F_hitch_body(1)*hHitch
    %Frz = (m*g*lf + m*ax_est*(h-hHitch) + Fz_hitch*(p_fax(1) - hitch(1)) ) / L; %+ F_hitch_body(1)*hHitch
    Ffz = (m*g*lr - m*ax_est*h + Fz_hitch*(hitch(1) - p_rax(1)) - F_hitch_body(1)*hHitch) / L;
    Frz = (m*g*lf + m*ax_est*h + Fz_hitch*(p_fax(1) - hitch(1)) + F_hitch_body(1)*hHitch) / L;
    
    Fy_f = -Cf*alpha_f*Ffz;
    Fy_r = -Cr*alpha_r*Frz;
    
    a_spec_x = (Fx_vehicle - Fy_f*sin(delta) - F_hitch_body(1))/m;
    
    a_spec_y = (Fy_f*cos(delta) + Fy_r - F_hitch_body(2))/m;
    
    dwz = (lf*Fy_f*cos(delta) - lr*Fy_r - lhitch*(F_hitch_body(2)))/Jz;
    
    a_imu = [a_spec_x; a_spec_y; 0] + cross(omega,cross(omega,Rcog)) + cross([0;0;dwz],Rcog);
    v_imu = v_cog + cross(omega,Rcog);
    
    omega_rl = (vx - wz * w_track/2) / Rwheel;
    omega_rr = (vx + wz * w_track/2) / Rwheel;
    omega_tr_ML = (v_tr_m(1) - wz_tr * w_track/2) / Rwheel;
    omega_tr_MR = (v_tr_m(1) + wz_tr * w_track/2) / Rwheel;
    
    % Z: [ax; ay; vx; vy; wz; w_rl; w_rr; w_tr_l; w_tr_r; Fyh]
    Z(:,k)=[a_imu(1:2); v_imu(1); v_imu(2); wz; omega_rl; omega_rr; omega_tr_ML; omega_tr_MR; Fyh_mod];
end
%% ===== REST
z_pred=zeros(10,1);
for k=1:nSPx
    w=(k==1)*W0+(k>1)*Wi;
    z_pred=z_pred+w*Z(:,k);
end
valid_idx=true(10,1);
valid_idx=valid_idx & ~isnan(z);
z_used=z(valid_idx);
z_pred_used=z_pred(valid_idx);
Z_used=Z(valid_idx,:);
R_used=R(valid_idx,valid_idx);
S_cov=zeros(length(z_used));
Pxz=zeros(n,length(z_used));
for k=1:nSPx
    w=(k==1)*W0+(k>1)*Wi;
    dz=Z_used(:,k)-z_pred_used;
    dx=X_post(:,k)-x_pred;
    S_cov=S_cov+w*(dz*dz');
    Pxz=Pxz+w*(dx*dz');
end
S_cov=S_cov+R_used;
K=Pxz/S_cov;
x=x_pred + K*(z_used - z_pred_used);
Pk=P_pred - K*S_cov*K';
Pk=(Pk+Pk')/2 + 1e-9*eye(n);
%% OUTPUT
xhat=x;
P=Pk;
dxdt=dxdt_model;
innovation=zeros(length(z),1);
innovation(valid_idx)=z_used - z_pred_used;
K_out=zeros(n,length(z));
K_out(:,valid_idx)=K;
S_out=zeros(length(z));
S_out(valid_idx,valid_idx)=S_cov;
z_pred_out=z_pred;
end

== matlab function generic_Truck_And_Trailer/TruckMaker/Two_TRack_Model/MATLAB Function ==
  data: z input; u input; xhat output; Q input; R input; Ts input; P output
function [xhat, P] = EKF_Bicycle_Full_NoBias(z, u, Q, R, Ts)
% EKF for One-Track / Bicycle Model (No IMU Bias)
% States: x = [vx; vy; r; Cf; Cr]
% Measurements: z = [ax; ay; vx; vy; r; wL; wR]

persistent x Pk
if isempty(x)
    % Initial state guess
    x = [15; 0; 0.05; 6e4; 6e4]; % vx, vy, r, Cf, Cr
    Pk = diag([1 1 0.05 2e4 2e4].^2);
end

%% Vehicle parameters
m  = 7000;       % mass
Jz = 14232;      % yaw inertia
lf = 1.12;       % front CG distance
lr = 2.45;       % rear CG distance
Rw = 0.49;       % wheel radius
track = 2.49;    % track width

%% Inputs
delta = u(1); % steering angle
Fx = u(2);    % longitudinal force

%% States
vx = x(1); vy = x(2); r = x(3);
Cf = x(4); Cr = x(5);

%% Protect low velocity
vx_eff = max(abs(vx), 3);

%% ---------------- Prediction ----------------
% Slip angles
alpha_f = (vy + lf*r)/vx_eff - delta;
alpha_r = (vy - lr*r)/vx_eff;

% Tire lateral forces
Fyf = -Cf*alpha_f; % Cyf= FyF/slip
Fyr = -Cr*alpha_r;

% Vehicle dynamics
dvx = (Fx - Fyf*sin(delta) + vy*r)/m;
dvy = (Fyf*cos(delta) + Fyr - vx*r)/m;
dr  = (lf*Fyf*cos(delta) - lr*Fyr)/Jz;

% State propagation
xdot = [dvx; dvy; dr; 0; 0];
x_pred = x + Ts*xdot;

%% ---------------- Jacobian F ----------------
F = eye(5);

% Partial derivatives for F
% alpha derivatives
dalf_dvx = -(vy + lf*r)/vx_eff^2;
dalf_dvy = 1/vx_eff;
dalf_dr  = lf/vx_eff;

dalr_dvx = -(vy - lr*r)/vx_eff^2;
dalr_dvy = 1/vx_eff;
dalr_dr  = -lr/vx_eff;

dFyf = -Cf*[dalf_dvx; dalf_dvy; dalf_dr];
dFyr = -Cr*[dalr_dvx; dalr_dvy; dalr_dr];

% dvx
F(1,1) = 1 + Ts*(-sin(delta)*dFyf(1))/m;
F(1,2) = Ts*(r - sin(delta)*dFyf(2))/m;
F(1,3) = Ts*(vy - sin(delta)*dFyf(3))/m;
F(1,4) = Ts*(-alpha_f*sin(delta))/m;

% dvy
F(2,1) = Ts*(-r + cos(delta)*dFyf(1) + dFyr(1))/m;
F(2,2) = 1 + Ts*(cos(delta)*dFyf(2) + dFyr(2))/m;
F(2,3) = Ts*( -vx + cos(delta)*dFyf(3) + dFyr(3))/m;
F(2,4) = Ts*(-alpha_f*cos(delta))/m;
F(2,5) = Ts*(-alpha_r)/m;

% dr
F(3,1) = Ts*(lf*cos(delta)*dFyf(1) - lr*dFyr(1))/Jz;
F(3,2) = Ts*(lf*cos(delta)*dFyf(2) - lr*dFyr(2))/Jz;
F(3,3) = 1 + Ts*(lf*cos(delta)*dFyf(3) - lr*dFyr(3))/Jz;
F(3,4) = Ts*(-lf*alpha_f*cos(delta))/Jz;
F(3,5) = Ts*(lr*alpha_r)/Jz;

%% ---------------- Covariance prediction ----------------
P_pred = F*Pk*F' + Q;

%% ---------------- Measurement model ----------------
ax_hat = dvx - vy*r;                % longitudinal accel
ay_hat = dvy + vx*r;                % lateral accel
vx_hat = vx;
vy_hat = vy;
r_hat  = r;
wL_hat = (vx - track/2 * r)/Rw;
wR_hat = (vx + track/2 * r)/Rw;

z_hat = [ax_hat; ay_hat; vx_hat; vy_hat; r_hat; wL_hat; wR_hat];

%% ---------------- Measurement Jacobian H ----------------
H = zeros(7,5);

% ax = dvx - vy*r
H(1,1) = 0; % optional: include dvx derivative
H(1,2) = -r;
H(1,3) = -vy;

% ay = dvy + vx*r
H(2,1) = r;
H(2,2) = 1;
H(2,3) = vx;
H(2,4) = -alpha_f*cos(delta)/m;
H(2,5) = -alpha_r/m;

% vx
H(3,1) = 1;

% vy
H(4,2) = 1;

% r
H(5,3) = 1;

% wheel speeds
H(6,1) = 1/Rw;
H(6,3) = -track/(2*Rw);

H(7,1) = 1/Rw;
H(7,3) = track/(2*Rw);

%% ---------------- EKF update ----------------
S = H*P_pred*H' + R;
K = P_pred*H'/S;

x = x_pred + K*(z - z_hat);
Pk = (eye(5) - K*H)*P_pred;

%% ---------------- Output ----------------
xhat = x;
P = Pk;

end
